simulink model "ModelWithBiasEstimation"  (R2020b)
settings: Solver=FixedStepAuto  StartTime=0.0  StopTime=12250  FixedStep=0.05  RelTol=1e-3
undefined symbols (not defined in the file or in its folder): sensor
libraries: GenericINSLibrary x2
settings Model: Creator=Damerius  LastModifiedBy=Scythe
settings DataIOCC: ReturnWorkspaceOutputs=off
settings DebuggingCC: InheritedTsInSrcMsg=none  ArithmeticOperatorsInVariantConditions=warning
settings SFSimCC: SimUseLocalCustomCode=off  CustomCodeUndefinedFunction=UseInterfaceOnly
settings RTWCC: RTWUseLocalCustomCode=off

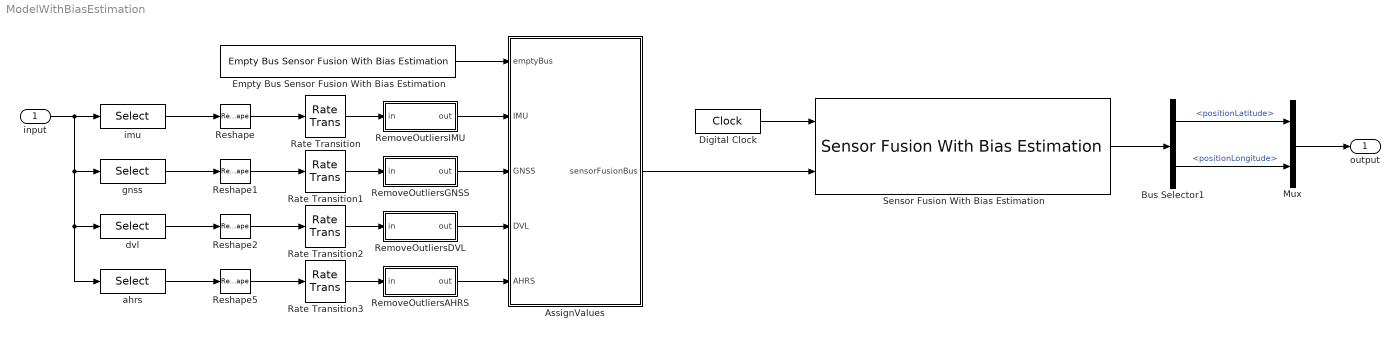
== system ModelWithBiasEstimation ==
  input : Inport
  AssignValues : Subsystem
  Bus Selector1 : BusSelector  OutputSignals=state.positionLatitude,state.positionLongitude
  Digital Clock : DigitalClock  SampleTime=0.05
  Empty Bus Sensor Fusion With Bias Estimation : GenericINSLibrary/Empty Bus Sensor Fusion With Bias Estimation
      settings: SourceProductName=Generic INS
  Mux : Mux  Inputs=2
  Rate Transition{,1..3} (4 alike) : RateTransition  Integrity=off  Deterministic=off  OutPortSampleTime=0.05
  RemoveOutliersAHRS : Subsystem
  RemoveOutliersDVL : Subsystem
  RemoveOutliersGNSS : Subsystem
  RemoveOutliersIMU : Subsystem
  Reshape : Reshape  OutputDimensionality=Customize  OutputDimensions=[7,1]
  Reshape1 : Reshape  OutputDimensionality=Customize  OutputDimensions=[4,1]
  Reshape2 : Reshape  OutputDimensionality=Customize  OutputDimensions=[4,1]
  Reshape5 : Reshape  OutputDimensionality=Customize  OutputDimensions=[4,1]
  Sensor Fusion With Bias Estimation : GenericINSLibrary/Sensor Fusion With Bias Estimation
      settings: SourceProductName=Generic INS
  ahrs : Selector  InputPortWidth=19  IndexOptions=Index vector (dialog)  Indices=16:19  OutputSizes=1
  dvl : Selector  InputPortWidth=19  IndexOptions=Index vector (dialog)  Indices=12:15  OutputSizes=1
  gnss : Selector  InputPortWidth=19  IndexOptions=Index vector (dialog)  Indices=8:11  OutputSizes=1
  imu : Selector  InputPortWidth=19  IndexOptions=Index vector (dialog)  Indices=1:7  OutputSizes=1
  output : Outport  VectorParamsAs1DForOutWhenUnconnected=off
  wires:
  input/1 -> imu/1, ahrs/1, dvl/1, gnss/1
  Mux/1 -> output/1
  Rate Transition1/1 -> RemoveOutliersGNSS/1(in)
  Rate Transition2/1 -> RemoveOutliersDVL/1(in)
  Rate Transition3/1 -> RemoveOutliersAHRS/1(in)
  ahrs/1 -> Reshape5/1
  Rate Transition/1 -> RemoveOutliersIMU/1(in)
  Digital Clock/1 -> Sensor Fusion With Bias Estimation/1
  Sensor Fusion With Bias Estimation/1 -> Bus Selector1/1
  Bus Selector1/1 -> Mux/1  "<positionLatitude>"
  Bus Selector1/2 -> Mux/2  "<positionLongitude>"
  Empty Bus Sensor Fusion With Bias Estimation/1 -> AssignValues/1(emptyBus)
  RemoveOutliersIMU/1(out) -> AssignValues/2(IMU)
  RemoveOutliersGNSS/1(out) -> AssignValues/3(GNSS)
  RemoveOutliersDVL/1(out) -> AssignValues/4(DVL)
  RemoveOutliersAHRS/1(out) -> AssignValues/5(AHRS)
  AssignValues/1(sensorFusionBus) -> Sensor Fusion With Bias Estimation/2
  Reshape5/1 -> Rate Transition3/1
  Reshape/1 -> Rate Transition/1
  imu/1 -> Reshape/1
  gnss/1 -> Reshape1/1
  dvl/1 -> Reshape2/1
  Reshape2/1 -> Rate Transition2/1
  Reshape1/1 -> Rate Transition1/1

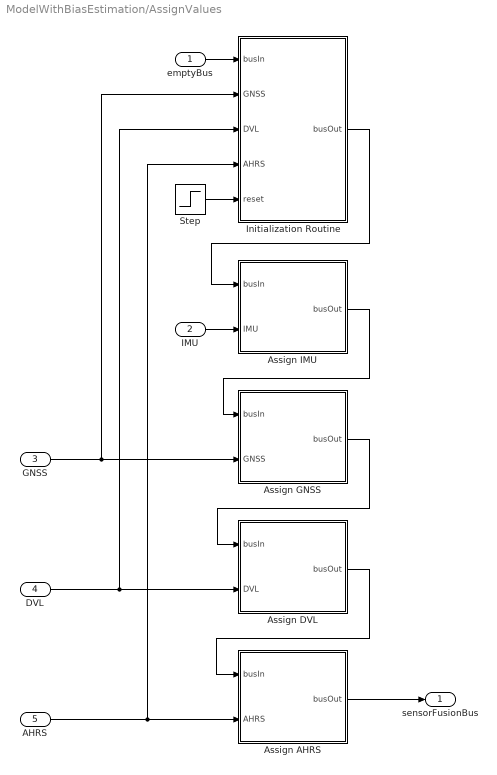
== system ModelWithBiasEstimation/AssignValues ==
  emptyBus : Inport
  IMU : Inport  Port=2
  GNSS : Inport  Port=3
  DVL : Inport  Port=4
  AHRS : Inport  Port=5
  Assign AHRS : Subsystem
  Assign DVL : Subsystem
  Assign GNSS : Subsystem
  Assign IMU : Subsystem
  Initialization Routine : Subsystem
  Step : Step  Time=0.05  Before=1  After=0
  sensorFusionBus : Outport
  wires:
  emptyBus/1 -> Initialization Routine/1(busIn)
  GNSS/1 -> Initialization Routine/2(GNSS), Assign GNSS/2(GNSS)
  DVL/1 -> Assign DVL/2(DVL), Initialization Routine/3(DVL)
  AHRS/1 -> Assign AHRS/2(AHRS), Initialization Routine/4(AHRS)
  Step/1 -> Initialization Routine/5(reset)
  Initialization Routine/1(busOut) -> Assign IMU/1(busIn)
  IMU/1 -> Assign IMU/2(IMU)
  Assign IMU/1(busOut) -> Assign GNSS/1(busIn)
  Assign GNSS/1(busOut) -> Assign DVL/1(busIn)
  Assign DVL/1(busOut) -> Assign AHRS/1(busIn)
  Assign AHRS/1(busOut) -> sensorFusionBus/1

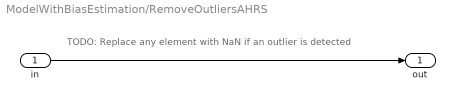
== system ModelWithBiasEstimation/RemoveOutliersAHRS ==
  note: TODO: Replace any element with NaN if an outlier is detected
  in : Inport
  out : Outport  VectorParamsAs1DForOutWhenUnconnected=off
  wires:
  in/1 -> out/1

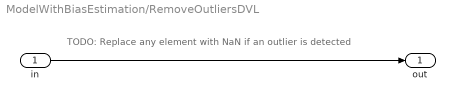
== system ModelWithBiasEstimation/RemoveOutliersDVL ==
  note: TODO: Replace any element with NaN if an outlier is detected
  in : Inport
  out : Outport  VectorParamsAs1DForOutWhenUnconnected=off
  wires:
  in/1 -> out/1

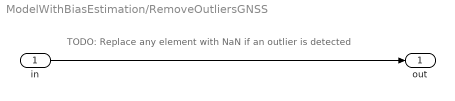
== system ModelWithBiasEstimation/RemoveOutliersGNSS ==
  note: TODO: Replace any element with NaN if an outlier is detected
  in : Inport
  out : Outport  VectorParamsAs1DForOutWhenUnconnected=off
  wires:
  in/1 -> out/1

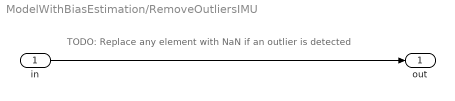
== system ModelWithBiasEstimation/RemoveOutliersIMU ==
  note: TODO: Replace any element with NaN if an outlier is detected
  in : Inport
  out : Outport  VectorParamsAs1DForOutWhenUnconnected=off
  wires:
  in/1 -> out/1

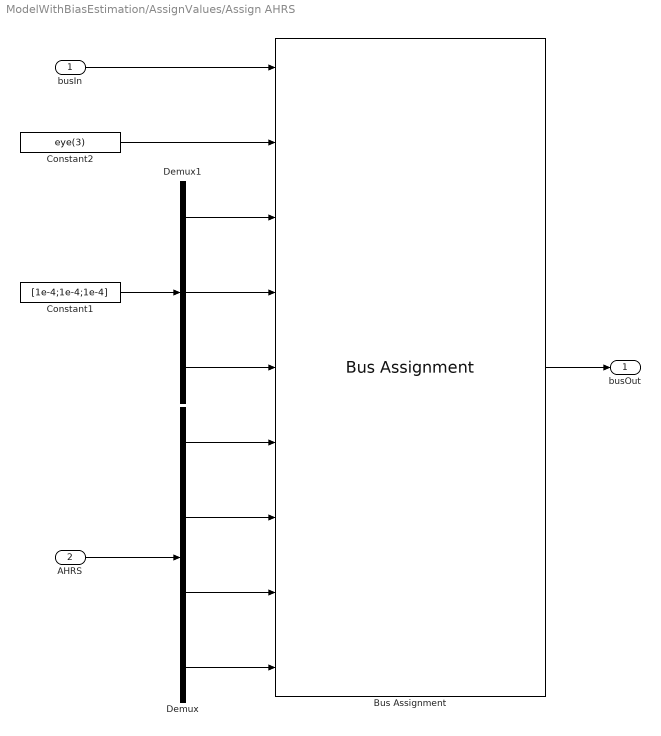
== system ModelWithBiasEstimation/AssignValues/Assign AHRS ==
  busIn : Inport
  AHRS : Inport  Port=2
  Bus Assignment : BusAssignment  AssignedSignals=sensor.AHRS1.alignment.rotationMatrixBodyToSensor,sensor.AHRS1.standardDeviation.roll,sensor.AHRS1.standardDeviation.pitch,sensor.AHRS1.standardDeviation.yaw,sensor.AHRS1.measurement.timestamp,sensor.AHRS1.measurement.roll,sensor.AHRS1.measurement.pitch,sensor.AHRS1.measurement.yaw
  Constant1 : Constant  Value=[1e-4;1e-4;1e-4]
  Constant2 : Constant  Value=eye(3)
  Demux : Demux
  Demux1 : Demux  Outputs=3
  busOut : Outport
  wires:
  AHRS/1 -> Demux/1
  busIn/1 -> Bus Assignment/1
  Bus Assignment/1 -> busOut/1
  Constant1/1 -> Demux1/1
  Constant2/1 -> Bus Assignment/2
  Demux1/3 -> Bus Assignment/5
  Demux1/2 -> Bus Assignment/4
  Demux1/1 -> Bus Assignment/3
  Demux/4 -> Bus Assignment/9
  Demux/3 -> Bus Assignment/8
  Demux/2 -> Bus Assignment/7
  Demux/1 -> Bus Assignment/6

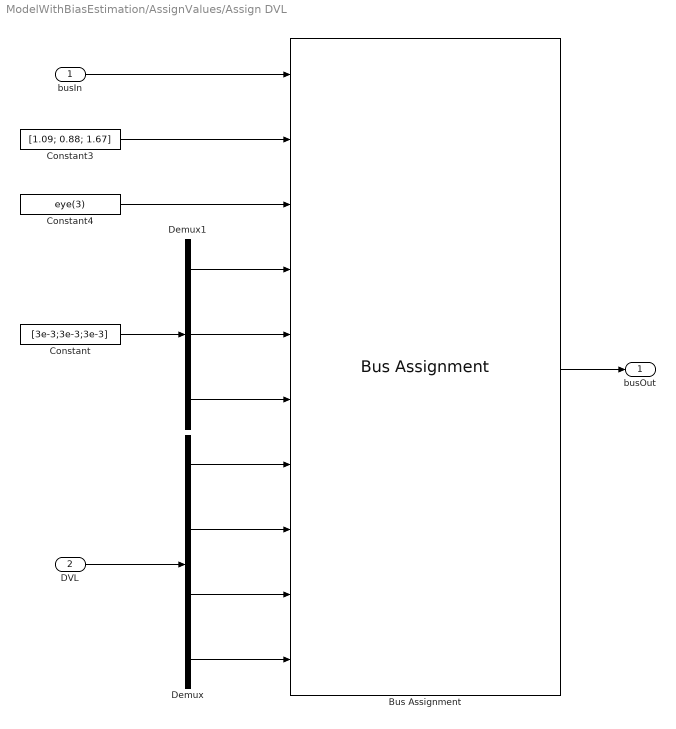
== system ModelWithBiasEstimation/AssignValues/Assign DVL ==
  busIn : Inport
  DVL : Inport  Port=2
  Bus Assignment : BusAssignment  AssignedSignals=sensor.VelocityXYZ1.alignment.positionBodyToSensor,sensor.VelocityXYZ1.alignment.rotationMatrixBodyToSensor,sensor.VelocityXYZ1.standardDeviation.velocityX,sensor.VelocityXYZ1.standardDeviation.velocityY,sensor.VelocityXYZ1.standardDeviation.velocityZ,sensor.VelocityXYZ1.measurement.timestamp,sensor.VelocityXYZ1.measurement.velocityX,sensor.VelocityXYZ1.measurement.velocityY,sensor.VelocityXYZ1.measurement.velocityZ
  Constant : Constant  Value=[3e-3;3e-3;3e-3]
  Constant3 : Constant  Value=[1.09; 0.88; 1.67]
  Constant4 : Constant  Value=eye(3)
  Demux : Demux
  Demux1 : Demux  Outputs=3
  busOut : Outport
  wires:
  Constant/1 -> Demux1/1
  Bus Assignment/1 -> busOut/1
  busIn/1 -> Bus Assignment/1
  DVL/1 -> Demux/1
  Constant3/1 -> Bus Assignment/2
  Constant4/1 -> Bus Assignment/3
  Demux1/1 -> Bus Assignment/4
  Demux1/2 -> Bus Assignment/5
  Demux1/3 -> Bus Assignment/6
  Demux/1 -> Bus Assignment/7
  Demux/2 -> Bus Assignment/8
  Demux/3 -> Bus Assignment/9
  Demux/4 -> Bus Assignment/10

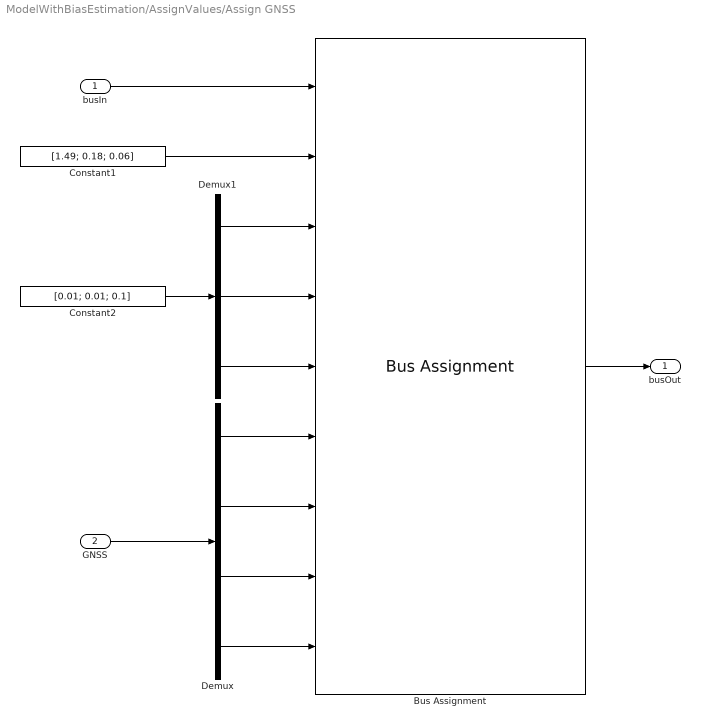
== system ModelWithBiasEstimation/AssignValues/Assign GNSS ==
  busIn : Inport
  GNSS : Inport  Port=2
  Bus Assignment : BusAssignment  AssignedSignals=sensor.GNSS1.alignment.positionBodyToSensor,sensor.GNSS1.standardDeviation.north,sensor.GNSS1.standardDeviation.east,sensor.GNSS1.standardDeviation.down,sensor.GNSS1.measurement.timestamp,sensor.GNSS1.measurement.latitude,sensor.GNSS1.measurement.longitude,sensor.GNSS1.measurement.altitude
  Constant1 : Constant  Value=[1.49; 0.18; 0.06]
  Constant2 : Constant  Value=[0.01; 0.01; 0.1]
  Demux : Demux
  Demux1 : Demux  Outputs=3
  busOut : Outport
  wires:
  GNSS/1 -> Demux/1
  busIn/1 -> Bus Assignment/1
  Bus Assignment/1 -> busOut/1
  Demux/4 -> Bus Assignment/9
  Demux/3 -> Bus Assignment/8
  Demux/2 -> Bus Assignment/7
  Demux/1 -> Bus Assignment/6
  Demux1/1 -> Bus Assignment/3
  Demux1/2 -> Bus Assignment/4
  Demux1/3 -> Bus Assignment/5
  Constant1/1 -> Bus Assignment/2
  Constant2/1 -> Demux1/1

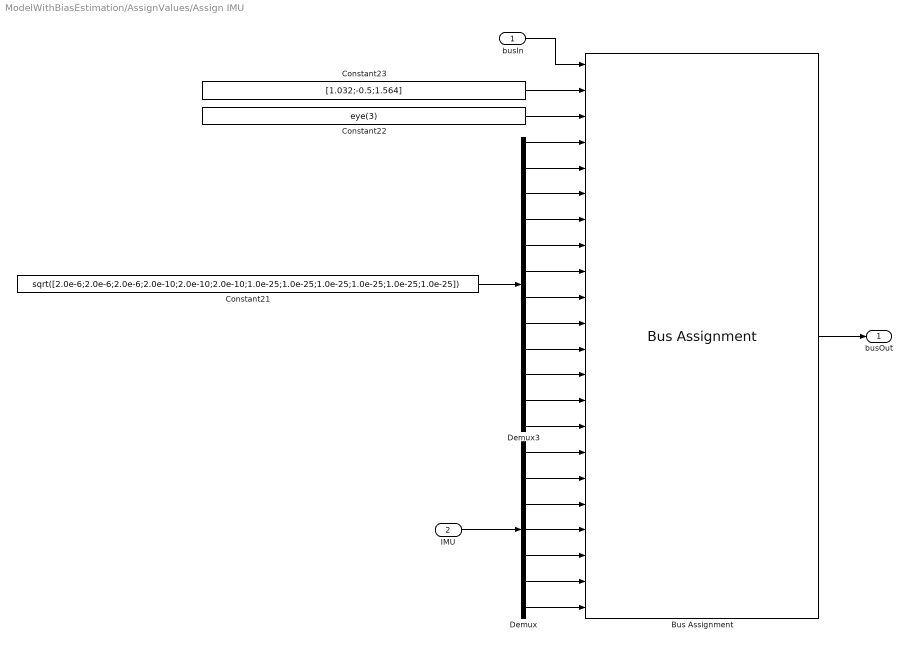
== system ModelWithBiasEstimation/AssignValues/Assign IMU ==
  busIn : Inport
  IMU : Inport  Port=2
  Bus Assignment : BusAssignment  AssignedSignals=sensor.IMU.alignment.positionBodyToSensor,sensor.IMU.alignment.rotationMatrixBodyToSensor,sensor.IMU.standardDeviation.accelerationX,sensor.IMU.standardDeviation.accelerationY,sensor.IMU.standardDeviation.accelerationZ,sensor.IMU.standardDeviation.angularRateX,sensor.IMU.standardDeviation.angularRateY,sensor.IMU.standardDeviation.angularRateZ,sensor.IMU.standardDeviation.biasAccelerationX,sensor.IMU.standardDeviation.biasAccelerationY,sensor.IMU.standardDeviation.biasAccelerationZ,sensor.IMU.standardDeviation.biasAngularRateX,sensor.IMU.standardDeviation.biasAngularRateY,sensor.IMU.standardDeviation.biasAngularRateZ,sensor.IMU.measurement.timestamp,sensor.IMU.measurement.accelerationX,sensor.IMU.measurement.accelerationY,sensor.IMU.measurement.accelerationZ,sensor.IMU.measurement.angularRateX,sensor.IMU.measurement.angularRateY,sensor.IMU.measurement.angularRateZ
  Constant21 : Constant  Value=sqrt([2.0e-6;2.0e-6;2.0e-6;2.0e-10;2.0e-10;2.0e-10;1.0e-25;1.0e-25;1.0e-25;1.0e-25;1.0e-25;1.0e-25])
  Constant22 : Constant  Value=eye(3)
  Constant23 : Constant  Value=[1.032;-0.5;1.564]
  Demux : Demux  Outputs=7
  Demux3 : Demux  Outputs=12
  busOut : Outport
  wires:
  Bus Assignment/1 -> busOut/1
  busIn/1 -> Bus Assignment/1
  IMU/1 -> Demux/1
  Constant23/1 -> Bus Assignment/2
  Constant22/1 -> Bus Assignment/3
  Demux3/9 -> Bus Assignment/12
  Demux3/10 -> Bus Assignment/13
  Demux3/8 -> Bus Assignment/11
  Demux3/11 -> Bus Assignment/14
  Demux3/7 -> Bus Assignment/10
  Demux3/12 -> Bus Assignment/15
  Demux3/6 -> Bus Assignment/9
  Demux3/5 -> Bus Assignment/8
  Demux3/4 -> Bus Assignment/7
  Demux3/3 -> Bus Assignment/6
  Demux3/2 -> Bus Assignment/5
  Demux3/1 -> Bus Assignment/4
  Constant21/1 -> Demux3/1
  Demux/3 -> Bus Assignment/18
  Demux/2 -> Bus Assignment/17
  Demux/4 -> Bus Assignment/19
  Demux/1 -> Bus Assignment/16
  Demux/5 -> Bus Assignment/20
  Demux/6 -> Bus Assignment/21
  Demux/7 -> Bus Assignment/22

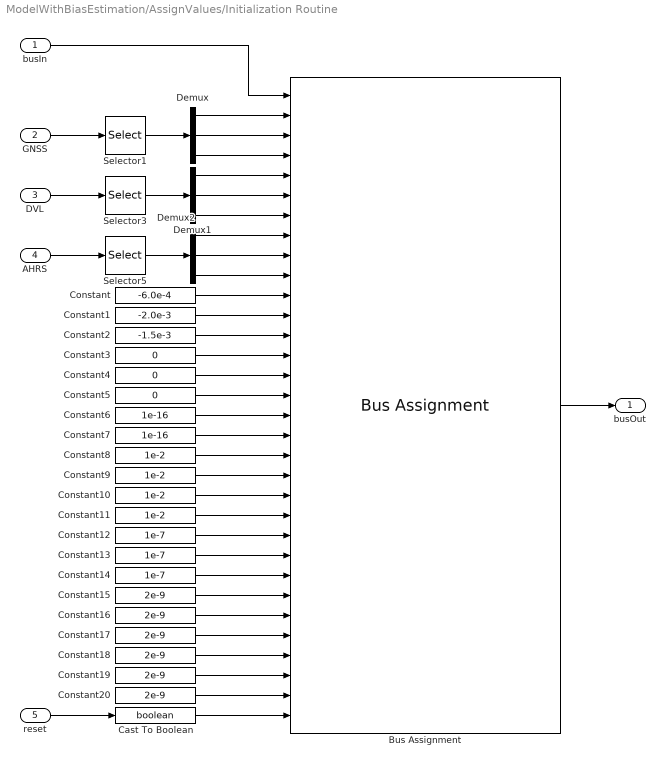
== system ModelWithBiasEstimation/AssignValues/Initialization Routine ==
  busIn : Inport
  GNSS : Inport  Port=2
  DVL : Inport  Port=3
  AHRS : Inport  Port=4
  reset : Inport  Port=5
  Bus Assignment : BusAssignment  AssignedSignals=initialization.initialState.latitude,initialization.initialState.longitude,initialization.initialState.altitude,initialization.initialState.velocityU,initialization.initialState.velocityV,initialization.initialState.velocityW,initialization.initialState.roll,initialization.initialState.pitch,initialization.initialState.yaw,initialization.initialState.biasAccelerationX,initialization.initialState.biasAccelerationY,initialization.initialState.biasAccelerationN,initialization.initialState.biasAngularRateX,initialization.initialState.biasAngularRateY,initialization.initialState.biasAngularRateZ,initialization.initialStandardDeviation.latitude,initialization.initialStandardDeviation.longitude,initialization.initialStandardDeviation.altitude,initialization.initialStandardDeviation.velocityU,initialization.initialStandardDeviation.velocityV,initialization.initialStandardDeviation.velocityW,initialization.initialStandardDeviation.orientationVectorX,initialization.initialStandardDeviation.orientationVectorY,initialization.initialStandardDeviation.orientationVectorZ,initialization.initialStandardDeviation.biasAccelerationX,initialization.initialStandardDeviation.biasAccelerationY,initialization.initialStandardDeviation.biasAccelerationN,initialization.initialStandardDeviation.biasAngularRateX,initialization.initialStandardDeviation.biasAngularRateY,initialization.initialStandardDeviation.biasAngularRateZ,initialization.reset
  Cast To Boolean : DataTypeConversion  OutDataTypeStr=boolean
  Constant : Constant  Value=-6.0e-4
  Constant1 : Constant  Value=-2.0e-3
  Constant{8..11} (4 alike) : Constant  Value=1e-2
  Constant12 : Constant  Value=1e-7
  Constant13 : Constant  Value=1e-7
  Constant14 : Constant  Value=1e-7
  Constant{15..20} (6 alike) : Constant  Value=2e-9
  Constant2 : Constant  Value=-1.5e-3
  Constant3 : Constant  Value=0
  Constant4 : Constant  Value=0
  Constant5 : Constant  Value=0
  Constant6 : Constant  Value=1e-16
  Constant7 : Constant  Value=1e-16
  Demux : Demux  Outputs=3
  Demux1 : Demux  Outputs=3
  Demux2 : Demux  Outputs=3
  Selector1 : Selector  InputPortWidth=4  IndexOptions=Index vector (dialog)  Indices=2:4  OutputSizes=1
  Selector3 : Selector  InputPortWidth=4  IndexOptions=Index vector (dialog)  Indices=2:4  OutputSizes=1
  Selector5 : Selector  InputPortWidth=4  IndexOptions=Index vector (dialog)  Indices=2:4  OutputSizes=1
  busOut : Outport
  wires:
  GNSS/1 -> Selector1/1
  DVL/1 -> Selector3/1
  AHRS/1 -> Selector5/1
  busIn/1 -> Bus Assignment/1
  Demux/2 -> Bus Assignment/3
  Demux/1 -> Bus Assignment/2
  Demux/3 -> Bus Assignment/4
  Selector1/1 -> Demux/1
  Demux1/3 -> Bus Assignment/7
  Demux1/2 -> Bus Assignment/6
  Demux1/1 -> Bus Assignment/5
  Selector3/1 -> Demux1/1
  Demux2/2 -> Bus Assignment/9
  Demux2/3 -> Bus Assignment/10
  Demux2/1 -> Bus Assignment/8
  Selector5/1 -> Demux2/1
  Constant/1 -> Bus Assignment/11
  Constant1/1 -> Bus Assignment/12
  Constant2/1 -> Bus Assignment/13
  Constant3/1 -> Bus Assignment/14
  Constant4/1 -> Bus Assignment/15
  Constant5/1 -> Bus Assignment/16
  Constant6/1 -> Bus Assignment/17
  Constant7/1 -> Bus Assignment/18
  Constant8/1 -> Bus Assignment/19
  Constant9/1 -> Bus Assignment/20
  Constant10/1 -> Bus Assignment/21
  Constant11/1 -> Bus Assignment/22
  Constant12/1 -> Bus Assignment/23
  Constant13/1 -> Bus Assignment/24
  Constant14/1 -> Bus Assignment/25
  Constant15/1 -> Bus Assignment/26
  Constant16/1 -> Bus Assignment/27
  Constant17/1 -> Bus Assignment/28
  Constant18/1 -> Bus Assignment/29
  Constant19/1 -> Bus Assignment/30
  Constant20/1 -> Bus Assignment/31
  reset/1 -> Cast To Boolean/1
  Bus Assignment/1 -> busOut/1
  Cast To Boolean/1 -> Bus Assignment/32
